simulink model "MPSK"  (R2017b)
settings: Solver=VariableStepAuto  StartTime=0.0  StopTime=1  RelTol=1e-3
values from neighbouring files (symbols this model uses):
  M = 2^K    (= 4)    [Digital_QAM.m]    (also in MPSK_constellation_decisionRegions.m; MPSK_frame_based_init.m = 2; MPSK_init.m = 2; MPSK_sample_based_init.m = 2)
  phaseOffset = pi    (= 3.14159265359)    [MPSK_frame_based_init.m]    (also in MPSK_init.m = -0.785398163397; MPSK_sample_based_init.m)
undefined symbols (not defined in the file or in its folder): i
libraries: commutil2 x2, commchan3 x1, simulink x1, commseqgen3 x1, commsink2 x1, commrflib2 x1, commrandsrc3 x1
settings Model: Creator=john3  LastModifiedBy=john3

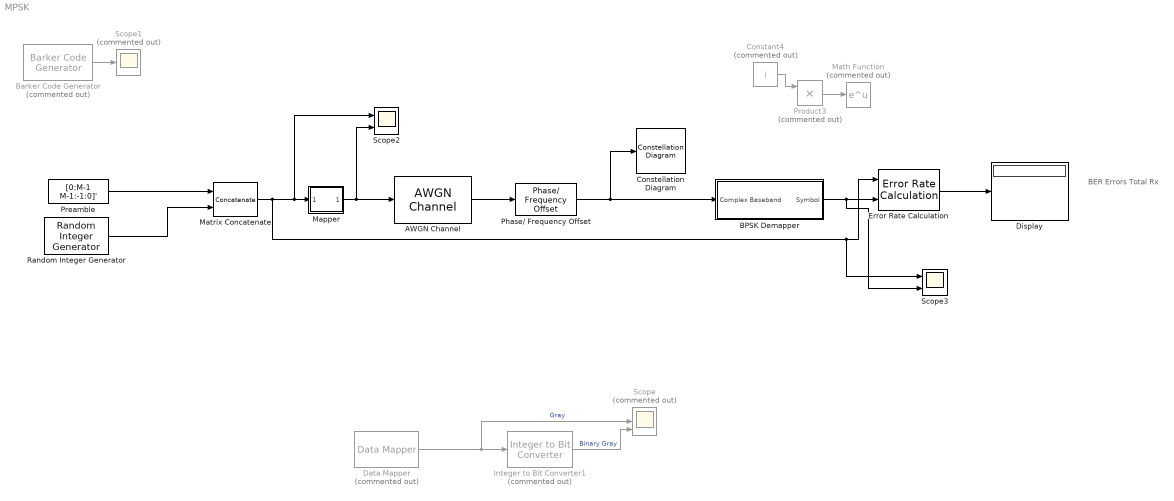
== system MPSK ==
  note: BER
      | Errors
      | Total Rx
  AWGN Channel : commchan3/AWGN Channel  InputProcessing=Columns as channels (frame based)  seed=67  noiseMode="Signal to noise ratio  (SNR)"  EbNodB=10  EsNodB=10  SNRdB=30  bitsPerSym=K  Ps=1  Tsym=1  variance=1
  BPSK Demapper : Subsystem
  Barker Code Generator : commseqgen3/Barker Code Generator  Commented=on  Length=7  LengthSimulink=7  SampleTime=1  SamplesPerFrame=1  OutputDataType=double  SimulateUsing=Interpreted execution
      settings: SourceProductName=Communications System Toolbox  SourceProductBaseCode=CM
  Constant4 : Constant  Commented=on  Value=i
  Constellation Diagram : ConstellationDiagram
  Data Mapper : commutil2/Data Mapper  Commented=on  MapMode=Binary to Gray  M=M  MapVec=[0 1 3 2 7 6 4 5]
      settings: SourceProductName=Communications System Toolbox  SourceProductBaseCode=CM
  Display : Display
  Error Rate Calculation : commsink2/Error Rate Calculation  N=0  st_delay=0  cp_mode=Entire frame  subframe=[]  PMode=Port  WsName=ErrorVec  RsMode2=off  stop=off  numErr=100  maxBits=1e6
  Integer to Bit Converter1 : commutil2/Integer to Bit Converter  Commented=on  nbits=K  signedInputValues=Unsigned  bitOrder=MSB first  outDtype=Inherit via internal rule
  Mapper : Subsystem
  Math Function : Math  Commented=on  SaturateOnIntegerOverflow=on
  Matrix Concatenate : Concatenate  Mode=Multidimensional array
  Phase/ Frequency Offset : commrflib2/Phase// Frequency Offset  phaseOffset=phaseOffset*180/pi  freqPort=off  freqOffset=0
      settings: SourceProductName=Communications System Toolbox
  Preamble : Constant  Value=[0:M-1 M-1:-1:0]'  SampleTime=1
  Product3 : Product  Commented=on
  Random Integer Generator : commrandsrc3/Random Integer Generator  SetSize=M  SeedSource=Auto  Seed=0  SampleTime=1/96  SamplesPerFrame=96  OutputDataType=double  SimulateUsing=Interpreted execution
  Scope : Scope  Commented=on  NumInputPorts=3
  Scope1 : Scope  Commented=on
  Scope2 : Scope  NumInputPorts=2
  Scope3 : Scope  NumInputPorts=2
  wires:
  Data Mapper/1 -> Scope/2, Integer to Bit Converter1/1  "Gray"
  Integer to Bit Converter1/1 -> Scope/3  "Binary Gray"
  AWGN Channel/1 -> Phase/ Frequency Offset/1
  Product3/1 -> Math Function/1
  Constant4/1 -> Product3/1
  Phase/ Frequency Offset/1 -> BPSK Demapper/1(Complex Baseband), Constellation Diagram/1
  BPSK Demapper/1(Symbol) -> Scope3/2, Error Rate Calculation/2
  Error Rate Calculation/1 -> Display/1
  Barker Code Generator/1 -> Scope1/1
  Preamble/1 -> Matrix Concatenate/1
  Random Integer Generator/1 -> Matrix Concatenate/2
  Matrix Concatenate/1 -> Scope3/1, Error Rate Calculation/1, Scope2/1, Mapper/1(In1)
  Mapper/1(Out1) -> Scope2/2, AWGN Channel/1

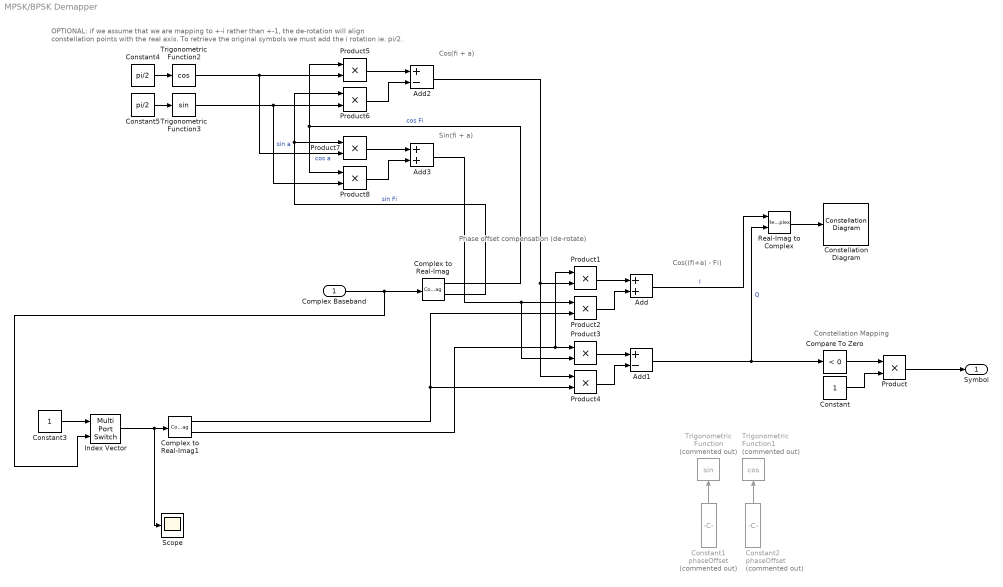
== system MPSK/BPSK Demapper ==
  note: OPTIONAL: if we assume that we are mapping to +-i rather than +-1, the de-rotation will align constellation points with the real axis.
      | To retrieve the original symbols we must add the i rotation ie. pi/2.
  note: Cos((fi+a) - Fi)
  note: Cos(fi + a)
  note: Phase offset compensation (de-rotate)
  note: Constellation Mapping
  note: Sin(fi + a)
  Complex Baseband : Inport
  Add : Sum
  Add1 : Sum  Inputs=+-
  Add2 : Sum  Inputs=+-
  Add3 : Sum
  Compare To Zero : simulink/Logic and Bit Operations/Compare To Zero  relop=<  OutDataTypeStr=boolean
  Complex to Real-Imag : ComplexToRealImag
  Complex to Real-Imag1 : ComplexToRealImag
  Constant : Constant
  Constant1 : Constant  Commented=on  Value=phaseOffset
  Constant2 : Constant  Commented=on  Value=phaseOffset
  Constant3 : Constant
  Constant4 : Constant  Value=pi/2
  Constant5 : Constant  Value=pi/2
  Constellation Diagram : ConstellationDiagram
  Index Vector : MultiPortSwitch  DataPortOrder=Zero-based contiguous  Inputs=1  zeroidx=on
  Product{,1..8} (9 alike) : Product
  Real-Imag to Complex : RealImagToComplex
  Scope : Scope
  Trigonometric Function : Trigonometry  Commented=on
  Trigonometric Function1 : Trigonometry  Commented=on  Operator=cos
  Trigonometric Function2 : Trigonometry  Operator=cos
  Trigonometric Function3 : Trigonometry
  Symbol : Outport
  wires:
  Compare To Zero/1 -> Product/1
  Complex Baseband/1 -> Index Vector/2, Complex to Real-Imag/1
  Constant/1 -> Product/2
  Constant1/1 -> Trigonometric Function/1
  Constant2/1 -> Trigonometric Function1/1
  Real-Imag to Complex/1 -> Constellation Diagram/1
  Product1/1 -> Add/1
  Product2/1 -> Add/2
  Product3/1 -> Add1/1
  Product4/1 -> Add1/2
  Complex to Real-Imag/1 -> Product5/1, Product8/1  "cos Fi"
  Add/1 -> Real-Imag to Complex/1  "I"
  Add1/1 -> Compare To Zero/1, Real-Imag to Complex/2  "Q"
  Product/1 -> Symbol/1
  Constant3/1 -> Index Vector/1
  Index Vector/1 -> Complex to Real-Imag1/1, Scope/1
  Complex to Real-Imag/2 -> Product7/1, Product6/1  "sin Fi"
  Constant4/1 -> Trigonometric Function2/1
  Constant5/1 -> Trigonometric Function3/1
  Product5/1 -> Add2/1
  Product6/1 -> Add2/2
  Complex to Real-Imag1/1 -> Product4/2, Product2/2
  Product8/1 -> Add3/2
  Product7/1 -> Add3/1
  Complex to Real-Imag1/2 -> Product3/1, Product1/1
  Trigonometric Function2/1 -> Product7/2, Product5/2  "cos a"
  Trigonometric Function3/1 -> Product8/2, Product6/2  "sin a"
  Add2/1 -> Product1/2, Product4/1
  Add3/1 -> Product3/2, Product2/1

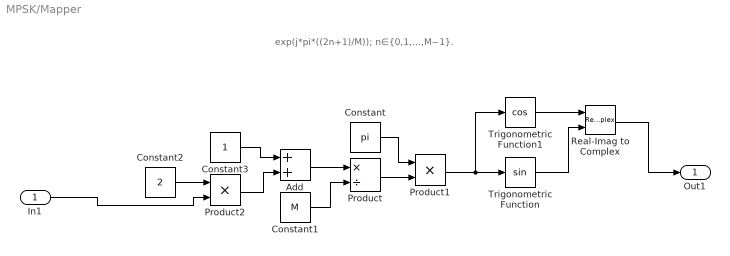
== system MPSK/Mapper ==
  note: exp(j*pi*((2n+1)/M)); n∈{0,1,…,M−1}.
  In1 : Inport
  Add : Sum
  Constant : Constant  Value=pi
  Constant1 : Constant  Value=M
  Constant2 : Constant  Value=2
  Constant3 : Constant
  Product : Product  Inputs=*/
  Product1 : Product
  Product2 : Product
  Real-Imag to Complex : RealImagToComplex
  Trigonometric Function : Trigonometry  ApproximationMethod=CORDIC
  Trigonometric Function1 : Trigonometry  Operator=cos  ApproximationMethod=CORDIC
  Out1 : Outport
  wires:
  Real-Imag to Complex/1 -> Out1/1
  Constant2/1 -> Product2/1
  In1/1 -> Product2/2
  Product1/1 -> Trigonometric Function1/1, Trigonometric Function/1
  Trigonometric Function1/1 -> Real-Imag to Complex/1
  Add/1 -> Product/1
  Product/1 -> Product1/2
  Constant3/1 -> Add/1
  Constant1/1 -> Product/2
  Trigonometric Function/1 -> Real-Imag to Complex/2
  Product2/1 -> Add/2
  Constant/1 -> Product1/1
